simulink model "termin2v6_vorgabe"  (Simulink 8.3)
settings: Solver=FixedStepDiscrete  SolverMode=SingleTasking  StartTime=0.0  StopTime=32000/8000  RelTol=1e-3  AbsTol=1e-6
undefined symbols (not defined in the file or in its folder): fCoeffsTP, get
libraries: dspsigops x5, dspxfrm3 x2, dspsnks4 x2, dspsrcs4 x1
settings Model: Creator=dsv1_4  LastModifiedBy=dsv1_5  ExtModeTrigMode=oneshot  ExtModeArmWhenConnect=off
settings DataIOCC: LimitDataPoints=off  SignalLoggingName=sigsOut
settings OptimizationCC: BooleanDataType=off  ExpressionDepthLimit=2147483647  InitFltsAndDblsToZero=on
settings DebuggingCC: SaveWithParameterizedLinksMsg=none  SignalResolutionControl=TryResolveAllWithWarning  SolverPrmCheckMsg=none  MultiTaskDSMMsg=warning  MultiTaskCondExecSysMsg=none  FcnCallInpInsideContextMsg=UseLocalSettings
settings HardwareCC: TargetUnknown=on
settings RTWCC: IncludeERTFirstTime=on
settings GRTTargetCC: TargetFcnLib=ansi_tfl_tmw.mat  ModelReferenceCompliant=off  MatFileLogging=off

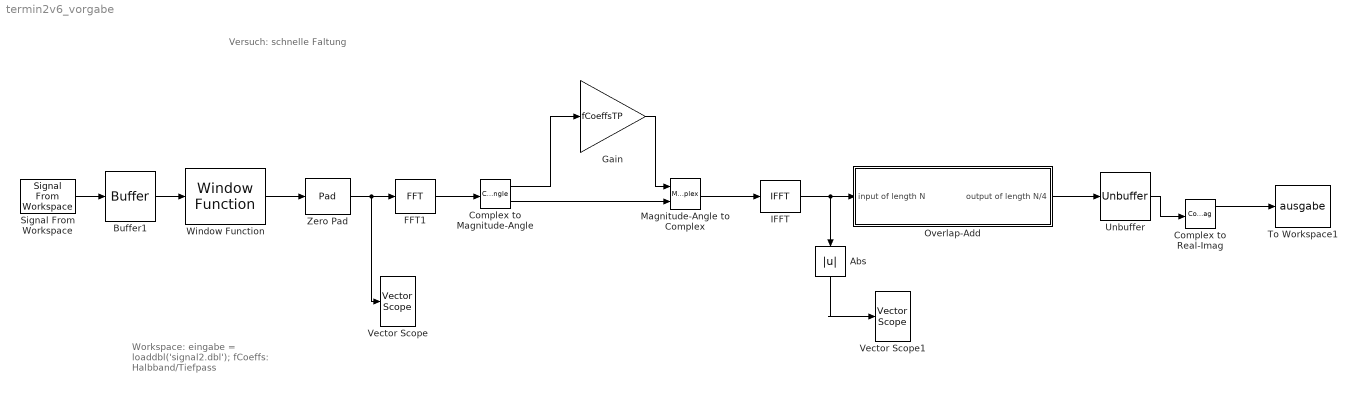
== system termin2v6_vorgabe ==
  note: Versuch: schnelle Faltung
  note: Workspace:
      | eingabe = loaddbl('signal2.dbl');
      | fCoeffs: Halbband/Tiefpass
  Abs : Abs
  Buffer1 : Buffer  N=256  V=128
  Complex to Magnitude-Angle : ComplexToMagnitudeAngle
  Complex to Real-Imag : ComplexToRealImag
  FFT1 : dspxfrm3/FFT  CompMethod=Table lookup  TableOpt=HYBRID  TableOptActive=Speed  BitRevOrder=off  InheritFFTLength=on  FFTLength=64  WrapInput=on  RowConvenienceOn=on  FFTImplementation=Auto  SkipNorm=off  firstCoeffDataTypeStr=Inherit: Same word length as input  firstCoeffLastDataTypeStr=Inherit: Same word length as input  outputMin=[]  outputMax=[]  roundingMode=Floor  overflowMode=off
  Gain : Gain  Gain=fCoeffsTP  SaturateOnIntegerOverflow=on  OutDataTypeStr=Inherit: Same as input  ParamDataTypeStr=Inherit: Same as input
  IFFT : dspxfrm3/IFFT  CompMethod=Table lookup  TableOpt=HYBRID  TableOptActive=Speed  BitRevOrder=off  cs_in=off  SkipNorm=on  InheritFFTLength=on  FFTLength=64  WrapInput=on  mode=Complex  outSamplingMode=Frame based  RowConvenienceOn=on  FFTImplementation=Auto  firstCoeffDataTypeStr=Inherit: Same word length as input  firstCoeffLastDataTypeStr=Inherit: Same word length as input  outputMin=[]  outputMax=[]  roundingMode=Floor  overflowMode=off
  Magnitude-Angle to Complex : MagnitudeAngleToComplex
  Overlap-Add : Subsystem
  Signal From Workspace : dspsrcs4/Signal From Workspace  X=signal2  Ts=1/8000  nsamps=1  OutputAfterFinalValue=Setting to zero  ignoreOrWarnInputAndFrameLengths=off
  To Workspace1 : ToWorkspace  VariableName=ausgabe  SampleTime=-1
      settings: MaxDataPoints=32000
  Unbuffer : Unbuffer
  Vector Scope : dspsnks4/Vector Scope  ScopeProperties=on  Domain=Time  HorizSpan=1  DisplayProperties=off  AxisGrid=on  Memory=off  FrameNumber=on  AxisLegend=off  AxisZoom=off  OpenScopeAtSimStart=on  OpenScopeImmediately=off  FigPos=get(0,'defaultfigureposition')  AxisProperties=off  XUnits=Hertz  XRange=[0...Fs/2]  InheritXIncr=on  XIncr=1  XLabel=Time  XLimit=Auto  XMin=0  XMax=1  XStart=0  YUnits=dB  YLabel=Amplitude  LineProperties=off  XAxisParamsVer=6.9
      settings: YMin=-10  YMax=10
  Vector Scope1 : dspsnks4/Vector Scope  ScopeProperties=on  Domain=Time  HorizSpan=1  DisplayProperties=off  AxisGrid=on  Memory=off  FrameNumber=on  AxisLegend=off  AxisZoom=off  OpenScopeAtSimStart=on  OpenScopeImmediately=off  FigPos=get(0,'defaultfigureposition')  AxisProperties=off  XUnits=Hertz  XRange=[0...Fs/2]  InheritXIncr=on  XIncr=1  XLabel=Time  XLimit=Auto  XMin=0  XMax=1  XStart=0  YUnits=dB  YLabel=Amplitude  LineProperties=off  XAxisParamsVer=6.9
      settings: YMin=-10  YMax=10
  Window Function : dspsigops/Window Function  winmode=Apply window to input  wintype=Hanning  sampmode=Continuous  samptime=1  N=1024  Rs=50  beta=10  winsamp=Symmetric  UserWindow=hamming  OptParams=off  UserParams={'symmetric'}  RowConvenienceOn=on  dataType=double  isSigned=on  wordLen=16  udDataType=sfix(16)  fracBitsMode=Best precision  numFracBits=15  roundingMode=Floor  overflowMode=off  numSidelobes=4  sidelobeLevel=-30
  Zero Pad : dspsigops/Pad  padAlong=Columns  dimsToPad=1  valSrc=Specify via dialog  padVal=0  spec=Output size  padNumOutRowsSpecMethod=User-specified  numOutRows=512  padNumOutColsSpecMethod=User-specified  numOutCols=1  isVarDimsMode=off  padBeginning=0  padEnd=0  outSizeMode=User-specified  outSize=1  padSigAt=End  trunc_flag=None  roundingMode=Floor  overflowMode=off  truncOrWrapMode=Truncate  wrap_flag=None
  wires:
  Signal From Workspace/1 -> Buffer1/1
  FFT1/1 -> Complex to Magnitude-Angle/1
  Window Function/1 -> Zero Pad/1
  Buffer1/1 -> Window Function/1
  Overlap-Add/1(output of length N/4) -> Unbuffer/1
  Zero Pad/1 -> Vector Scope/1, FFT1/1
  Gain/1 -> Magnitude-Angle to Complex/1
  IFFT/1 -> Abs/1, Overlap-Add/1(input of length N)
  Magnitude-Angle to Complex/1 -> IFFT/1
  Complex to Magnitude-Angle/1 -> Gain/1
  Complex to Magnitude-Angle/2 -> Magnitude-Angle to Complex/2
  Unbuffer/1 -> Complex to Real-Imag/1
  Complex to Real-Imag/1 -> To Workspace1/1
  Abs/1 -> Vector Scope1/1

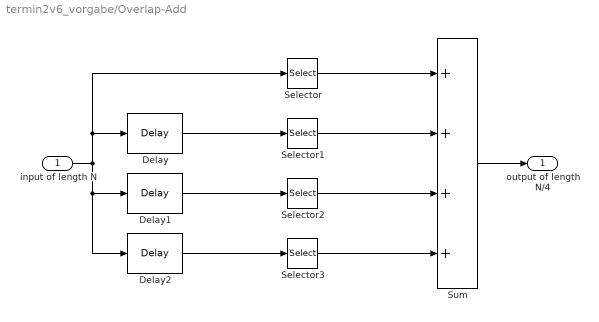
== system termin2v6_vorgabe/Overlap-Add ==
  input of length N : Inport
  Delay : dspsigops/Delay  InputProcessing=Inherited (this choice will be removed - see release notes)  dly_unit=Frames  delay=1  ic_detail=off  dif_ic_for_ch=off  dif_ic_for_dly=off  ic=0  reset_popup=None
  Delay1 : dspsigops/Delay  InputProcessing=Inherited (this choice will be removed - see release notes)  dly_unit=Frames  delay=2  ic_detail=off  dif_ic_for_ch=off  dif_ic_for_dly=off  ic=0  reset_popup=None
  Delay2 : dspsigops/Delay  InputProcessing=Inherited (this choice will be removed - see release notes)  dly_unit=Frames  delay=3  ic_detail=off  dif_ic_for_ch=off  dif_ic_for_dly=off  ic=0  reset_popup=None
  Selector : Selector  InputPortWidth=512  Indices=[1:128]
  Selector1 : Selector  InputPortWidth=512  Indices=[129:256]
  Selector2 : Selector  InputPortWidth=512  Indices=[257:384]
  Selector3 : Selector  InputPortWidth=512  Indices=[385:512]
  Sum : Sum  Inputs=++++  SaturateOnIntegerOverflow=on  InputSameDT=on  OutDataTypeStr=Inherit: Same as first input
  output of length N/4 : Outport  InitialOutput=0
  wires:
  Delay/1 -> Selector1/1
  Delay2/1 -> Selector3/1
  Selector/1 -> Sum/1
  Selector1/1 -> Sum/2
  Selector2/1 -> Sum/3
  Selector3/1 -> Sum/4
  Delay1/1 -> Selector2/1
  input of length N/1 -> Selector/1, Delay/1, Delay1/1, Delay2/1
  Sum/1 -> output of length N/4/1
